simulink model "RobotAndBall"  (R2019b)
settings: Solver=VariableStepAuto  StartTime=0.0  StopTime=30  MaxStep=updateFrequency  RelTol=1e-3
values from neighbouring files (symbols this model uses):
  g = bTraj.GoalOnRight    [Launch_Game_TwoRobots.m]
  pOpponentSidePoint = [2.4;0;0.02]'    [Launch_Game_TwoRobots.m]
  Robot1 = RobotPlayer2(initialQ,TransMat1,DistToTable,'Left')    [Launch_Game_TwoRobots.m]
undefined symbols (not defined in the file or in its folder): Ball, Contact_Forces, currentTime, Environment, Net, Robots, Table, tHit, wayPoints, X, Y, Z
libraries: sm_lib x217, nesl_utility x89, Contact_Forces_Lib x8, robotmaniplib x8, Parts_Lib x6, Multibody_Parts_Lib x2, OpenManipulatorLib x1
(part 7 of 7)

== system RobotAndBall/Subsystem2/Robot 2/Robotic Arm1/iiwa_link_7 ==
  Inertia : sm_lib/Body Elements/Inertia  InertiaType=Custom  Mass=3.129  MassUnits=kg  CenterOfMass=[0, 0, 0]  CenterOfMassUnits=m  MomentsOfInertia=[0.01464, 0.01465, 0.002872]  MomentsOfInertiaUnits=kg*m^2  ProductsOfInertia=[0, 0, 0.0005912]  ProductsOfInertiaUnits=kg*m^2  GraphicType=None  MarkerShape=Inertia  MarkerSize=20  GraphicVisPropType=SimpleVisualProperties  GraphicDiffuseColor=[0.5 0.5 0.5]  GraphicSpecularColor=[0.5 0.5 0.5 1.0]  GraphicAmbientColor=[0.15 0.15 0.15 1.0]  GraphicEmissiveColor=[0.0 0.0 0.0 1.0]  GraphicShininess=75  GraphicOpacity=1.0
  InertiaOriginTransform : sm_lib/Frames and Transforms/Rigid Transform  TranslationMethod=Cartesian  TranslationStandardOffset=0  TranslationLengthUnit=m  TranslationStandardAxis=+Z  TranslationCartesianOffset=[0, 0, 0.02]  TranslationROffset=0  TranslationROffsetUnits=m  TranslationZOffset=0  TranslationZOffsetUnits=m  TranslationThetaOffset=0  TranslationThetaOffsetUnits=deg  RotationMethod=RotationSequence  RotationAngleUnits=deg  RotationStandardAxis=+Z  RotationAngle=0.0  RotationArbitraryAxis=[0 0 1]  FollAlignAxisA=+X  BaseAlignAxisA=+Y  FollAlignAxisB=+Y  BaseAlignAxisB=+Z  RotationSequenceAxes=BaseAxes  RotationSequence=XYZ  RotationSequenceAngles=[0, 0, 0]  RotationSequenceAnglesUnits=rad  RotationMatrix=[1 0 0; 0 1 0; 0 0 1]
  ReferenceFrame : sm_lib/Frames and Transforms/Reference Frame
  Visual : sm_lib/Body Elements/File Solid  ExtGeomFileName=link_7.stl  UnitType=Custom  ExtGeomFileUnits=m  StepReaderType=HEX  ExportEntireGeometry=off  InertiaType=Custom  Mass=0  MassUnits=kg  CenterOfMass=[0, 0, 0]  CenterOfMassUnits=m  MomentsOfInertia=[0, 0, 0]  MomentsOfInertiaUnits=kg*m^2  ProductsOfInertia=[0, 0, 0]  ProductsOfInertiaUnits=kg*m^2  BasedOnType=DensityFromFile  Density=1000  DensityUnits=kg/m^3  DoExposeReferenceFrame=on  SerializedFrames=<Frames/>  GraphicType=FromGeometry  MarkerShape=Sphere  MarkerSize=10  GraphicVisPropType=SimpleVisualProperties  GraphicDiffuseColor=[0.4, 0.4, 0.4]  GraphicSpecularColor=[0.5 0.5 0.5 1.0]  GraphicAmbientColor=[0.15 0.15 0.15 1.0]  GraphicEmissiveColor=[0.0 0.0 0.0 1.0]  GraphicShininess=75  GraphicOpacity=1
  VisualOriginTransform : sm_lib/Frames and Transforms/Rigid Transform  TranslationMethod=Cartesian  TranslationStandardOffset=0  TranslationLengthUnit=m  TranslationStandardAxis=+Z  TranslationCartesianOffset=[0, 0, -0.0005]  TranslationROffset=0  TranslationROffsetUnits=m  TranslationZOffset=0  TranslationZOffsetUnits=m  TranslationThetaOffset=0  TranslationThetaOffsetUnits=deg  RotationMethod=RotationSequence  RotationAngleUnits=deg  RotationStandardAxis=+Z  RotationAngle=0.0  RotationArbitraryAxis=[0 0 1]  FollAlignAxisA=+X  BaseAlignAxisA=+Y  FollAlignAxisB=+Y  BaseAlignAxisB=+Z  RotationSequenceAxes=BaseAxes  RotationSequence=XYZ  RotationSequenceAngles=[0, 0, 0]  RotationSequenceAnglesUnits=rad  RotationMatrix=[1 0 0; 0 1 0; 0 0 1]
  iiwa_joint_7_AxisInvTransform : sm_lib/Frames and Transforms/Rigid Transform  TranslationMethod=Cartesian  TranslationStandardOffset=0  TranslationLengthUnit=m  TranslationStandardAxis=+Z  TranslationCartesianOffset=[0, 0, 0]  TranslationROffset=0  TranslationROffsetUnits=m  TranslationZOffset=0  TranslationZOffsetUnits=m  TranslationThetaOffset=0  TranslationThetaOffsetUnits=deg  RotationMethod=ArbitraryAxis  RotationAngleUnits=rad  RotationStandardAxis=+Z  RotationAngle=0  RotationArbitraryAxis=[1, 0, 0]  FollAlignAxisA=+X  BaseAlignAxisA=+Y  FollAlignAxisB=+Y  BaseAlignAxisB=+Z  RotationSequenceAxes=FollowerAxes  RotationSequence=XYX  RotationSequenceAngles=[0 0 0]  RotationSequenceAnglesUnits=deg  RotationMatrix=[1 0 0; 0 1 0; 0 0 1]
  iiwa_joint_8_AxisInvTransform1 : sm_lib/Frames and Transforms/Rigid Transform  TranslationMethod=Cartesian  TranslationStandardOffset=0  TranslationLengthUnit=m  TranslationStandardAxis=+Z  TranslationCartesianOffset=[0, 0, 0]  TranslationROffset=0  TranslationROffsetUnits=m  TranslationZOffset=0  TranslationZOffsetUnits=m  TranslationThetaOffset=0  TranslationThetaOffsetUnits=deg  RotationMethod=ArbitraryAxis  RotationAngleUnits=rad  RotationStandardAxis=+Z  RotationAngle=0  RotationArbitraryAxis=[0, 0, 1]  FollAlignAxisA=+X  BaseAlignAxisA=+Y  FollAlignAxisB=+Y  BaseAlignAxisB=+Z  RotationSequenceAxes=FollowerAxes  RotationSequence=XYX  RotationSequenceAngles=[0 0 0]  RotationSequenceAnglesUnits=deg  RotationMatrix=[1 0 0; 0 1 0; 0 0 1]
  iiwa_joint_ee_OriginTransform : sm_lib/Frames and Transforms/Rigid Transform  TranslationMethod=Cartesian  TranslationStandardOffset=0  TranslationLengthUnit=m  TranslationStandardAxis=+Z  TranslationCartesianOffset=[0, 0, 0.045]  TranslationROffset=0  TranslationROffsetUnits=m  TranslationZOffset=0  TranslationZOffsetUnits=m  TranslationThetaOffset=0  TranslationThetaOffsetUnits=deg  RotationMethod=RotationSequence  RotationAngleUnits=deg  RotationStandardAxis=+Z  RotationAngle=0.0  RotationArbitraryAxis=[0 0 1]  FollAlignAxisA=+X  BaseAlignAxisA=+Y  FollAlignAxisB=+Y  BaseAlignAxisB=+Z  RotationSequenceAxes=BaseAxes  RotationSequence=XYZ  RotationSequenceAngles=[0, 0, 0]  RotationSequenceAnglesUnits=rad  RotationMatrix=[1 0 0; 0 1 0; 0 0 1]
  F : PMIOPort  Side=Left
  F1 : PMIOPort  Port=2  Side=Right
  connections:
  Inertia/RConn1 -- InertiaOriginTransform/RConn1
  ReferenceFrame/RConn1 -- InertiaOriginTransform/LConn1 -- iiwa_joint_ee_OriginTransform/LConn1 -- iiwa_joint_7_AxisInvTransform/LConn1 -- VisualOriginTransform/LConn1
  Visual/RConn1 -- VisualOriginTransform/RConn1
  iiwa_joint_7_AxisInvTransform/RConn1 -- F/RConn1
  iiwa_joint_8_AxisInvTransform1/RConn1 -- F1/RConn1
  iiwa_joint_ee_OriginTransform/RConn1 -- iiwa_joint_8_AxisInvTransform1/LConn1

== system RobotAndBall/Subsystem2/Robot 2/Robotic Arm1/iiwa_link_8 ==
  Inertia : sm_lib/Body Elements/Inertia  InertiaType=Custom  Mass=0.24*0  MassUnits=kg  CenterOfMass=[0, 0, 0.02]*0  CenterOfMassUnits=m  MomentsOfInertia=[322.661e-6 , 1182.846e-6, 867.899e-6]*0  MomentsOfInertiaUnits=kg*m^2  ProductsOfInertia=[-0.001e-6, 0.002e-6, 0.021e-6]*0  ProductsOfInertiaUnits=kg*m^2  GraphicType=None  MarkerShape=Inertia  MarkerSize=20  GraphicVisPropType=SimpleVisualProperties  GraphicDiffuseColor=[0.5 0.5 0.5]  GraphicSpecularColor=[0.5 0.5 0.5 1.0]  GraphicAmbientColor=[0.15 0.15 0.15 1.0]  GraphicEmissiveColor=[0.0 0.0 0.0 1.0]  GraphicShininess=75  GraphicOpacity=1.0
  Inertia1 : sm_lib/Body Elements/Inertia  Commented=on  InertiaType=Custom  Mass=1000  MassUnits=kg  CenterOfMass=[0, 0, 0.02]  CenterOfMassUnits=m  MomentsOfInertia=1000*[322.661e-6 , 1182.846e-6, 867.899e-6]  MomentsOfInertiaUnits=kg*m^2  ProductsOfInertia=[-0.001e-6, 0.002e-6, 0.021e-6]  ProductsOfInertiaUnits=kg*m^2  GraphicType=None  MarkerShape=Inertia  MarkerSize=20  GraphicVisPropType=SimpleVisualProperties  GraphicDiffuseColor=[0.5 0.5 0.5]  GraphicSpecularColor=[0.5 0.5 0.5 1.0]  GraphicAmbientColor=[0.15 0.15 0.15 1.0]  GraphicEmissiveColor=[0.0 0.0 0.0 1.0]  GraphicShininess=75  GraphicOpacity=1.0
  InertiaOriginTransform : sm_lib/Frames and Transforms/Rigid Transform  TranslationMethod=Cartesian  TranslationStandardOffset=0  TranslationLengthUnit=m  TranslationStandardAxis=+Z  TranslationCartesianOffset=[0, 0,0.05]  TranslationROffset=0  TranslationROffsetUnits=m  TranslationZOffset=0  TranslationZOffsetUnits=m  TranslationThetaOffset=0  TranslationThetaOffsetUnits=deg  RotationMethod=RotationSequence  RotationAngleUnits=deg  RotationStandardAxis=+Z  RotationAngle=0.0  RotationArbitraryAxis=[0 0 1]  FollAlignAxisA=+X  BaseAlignAxisA=+Y  FollAlignAxisB=+Y  BaseAlignAxisB=+Z  RotationSequenceAxes=BaseAxes  RotationSequence=XYZ  RotationSequenceAngles=[0, 0, 0]  RotationSequenceAnglesUnits=rad  RotationMatrix=[1 0 0; 0 1 0; 0 0 1]
  ReferenceFrame : sm_lib/Frames and Transforms/Reference Frame
  Visual : sm_lib/Body Elements/File Solid  ExtGeomFileName=paddle.stl  UnitType=Custom  ExtGeomFileUnits=cm  StepReaderType=HEX  ExportEntireGeometry=off  InertiaType=Custom  Mass=0  MassUnits=kg  CenterOfMass=[0, 0, 0]  CenterOfMassUnits=m  MomentsOfInertia=[0, 0, 0]  MomentsOfInertiaUnits=kg*m^2  ProductsOfInertia=[0, 0, 0]  ProductsOfInertiaUnits=kg*m^2  BasedOnType=DensityFromFile  Density=1000  DensityUnits=kg/m^3  DoExposeReferenceFrame=on  SerializedFrames=<Frames/>  GraphicType=FromGeometry  MarkerShape=Sphere  MarkerSize=10  GraphicVisPropType=SimpleVisualProperties  GraphicDiffuseColor=[1, 0.423529411765, 0.0392156862745]  GraphicSpecularColor=[0.5 0.5 0.5 1.0]  GraphicAmbientColor=[0.15 0.15 0.15 1.0]  GraphicEmissiveColor=[0.0 0.0 0.0 1.0]  GraphicShininess=75  GraphicOpacity=1
  VisualOriginTransform : sm_lib/Frames and Transforms/Rigid Transform  TranslationMethod=Cartesian  TranslationStandardOffset=0  TranslationLengthUnit=m  TranslationStandardAxis=+Z  TranslationCartesianOffset=[0, 0, 0.12]  TranslationROffset=0  TranslationROffsetUnits=m  TranslationZOffset=0  TranslationZOffsetUnits=m  TranslationThetaOffset=0  TranslationThetaOffsetUnits=deg  RotationMethod=RotationSequence  RotationAngleUnits=deg  RotationStandardAxis=+Z  RotationAngle=0.0  RotationArbitraryAxis=[0 0 1]  FollAlignAxisA=+X  BaseAlignAxisA=+Y  FollAlignAxisB=+Y  BaseAlignAxisB=+Z  RotationSequenceAxes=BaseAxes  RotationSequence=XYZ  RotationSequenceAngles=[180, 0, 0]  RotationSequenceAnglesUnits=deg  RotationMatrix=[1 0 0; 0 1 0; 0 0 1]
  iiwa_joint_6_AxisInvTransform : sm_lib/Frames and Transforms/Rigid Transform  TranslationMethod=Cartesian  TranslationStandardOffset=0  TranslationLengthUnit=m  TranslationStandardAxis=+Z  TranslationCartesianOffset=[0, 0, 0]  TranslationROffset=0  TranslationROffsetUnits=m  TranslationZOffset=0  TranslationZOffsetUnits=m  TranslationThetaOffset=0  TranslationThetaOffsetUnits=deg  RotationMethod=ArbitraryAxis  RotationAngleUnits=rad  RotationStandardAxis=+Z  RotationAngle=0  RotationArbitraryAxis=[1, 0, 0]  FollAlignAxisA=+X  BaseAlignAxisA=+Y  FollAlignAxisB=+Y  BaseAlignAxisB=+Z  RotationSequenceAxes=FollowerAxes  RotationSequence=XYX  RotationSequenceAngles=[0 0 0]  RotationSequenceAnglesUnits=deg  RotationMatrix=[1 0 0; 0 1 0; 0 0 1]
  F : PMIOPort  Side=Left
  F1 : PMIOPort  Port=2  Side=Left
  connections:
  iiwa_joint_6_AxisInvTransform/RConn1 -- F/RConn1
  Visual/RConn1 -- F1/RConn1 -- VisualOriginTransform/RConn1
  VisualOriginTransform/LConn1 -- iiwa_joint_6_AxisInvTransform/LConn1 -- InertiaOriginTransform/LConn1 -- ReferenceFrame/RConn1
  Inertia/RConn1 -- InertiaOriginTransform/RConn1

== system RobotAndBall/Subsystem2/Robot 2/Robotic Arm1/world ==
  ReferenceFrame : sm_lib/Frames and Transforms/Reference Frame
  world_iiwa_joint_OriginTransform : sm_lib/Frames and Transforms/Rigid Transform  TranslationMethod=Cartesian  TranslationStandardOffset=0  TranslationLengthUnit=m  TranslationStandardAxis=+Z  TranslationCartesianOffset=[0, 0, 0]  TranslationROffset=0  TranslationROffsetUnits=m  TranslationZOffset=0  TranslationZOffsetUnits=m  TranslationThetaOffset=0  TranslationThetaOffsetUnits=deg  RotationMethod=RotationSequence  RotationAngleUnits=deg  RotationStandardAxis=+Z  RotationAngle=0.0  RotationArbitraryAxis=[0 0 1]  FollAlignAxisA=+X  BaseAlignAxisA=+Y  FollAlignAxisB=+Y  BaseAlignAxisB=+Z  RotationSequenceAxes=BaseAxes  RotationSequence=XYZ  RotationSequenceAngles=[0, 0, 0]  RotationSequenceAnglesUnits=rad  RotationMatrix=[1 0 0; 0 1 0; 0 0 1]
  F : PMIOPort  Side=Left
  F1 : PMIOPort  Port=2  Side=Right
  connections:
  world_iiwa_joint_OriginTransform/LConn1 -- ReferenceFrame/RConn1 -- F/RConn1
  world_iiwa_joint_OriginTransform/RConn1 -- F1/RConn1

== matlab function RobotAndBall/failTryToPredictTraj/MATLAB Function ==
  data: P input; aa output; V input; N input; t input
function aa = fcn(P,V,N,t)
%         if LastV(3)*V(3)<0 & V(3)>0
% %             Ball.N=0;
%                i = i+1
% %             set_param('Table_Ball','SimulationCommand','pause')
%         end
%         Ball.N=Ball.N+1;
%         Ball.Postitions(Ball.N,:)=P;
%         Ball.Velocities(Ball.N,:)=V;
        moments = (0:t/N:t) 
        if(N>5)
            [fitz,Predicted_P] = Traj_Predict(moments,P(1:N,:),N);
        end
        if Ball.N == 150
            figure 
            plot(fitz) ;
            aa = fitz.a
            fitz.b
            fitz.c
        end
%     end


LastP=P;
LastV=V;
y = u;

== matlab function RobotAndBall/Subsystem2/Air_resistance_Force ==
  data: wx input; f output; wy input; wz input; vx input; vy input; vz input; Cd input; Cl input
function f = Air_Resisctance_Force(wx,wy,wz,vx,vy,vz,Cd,Cl)
w = [wx;wy;wz];
v = [vx;vy;vz];
mb = 0.0027; % ball mass = 2.7 gram
% Cd = Environment.AirDrag;%0.141   ; % drag coefficient
% Cl = Environment.Magnus%0.001; % Magnus coefficient
% Cd = 1;
%a = g - Cd*|v|*v + Cl*(w x b)
f = mb*(-Cd*norm(v)*v + Cl*cross(w,v));

== matlab function RobotAndBall/failTryToPredictTraj/Append ==
  data: V input; Vnew input; P input; Pout output; Vout output; Pnew input; N input; Nout output
function [Pout,Vout,Nout]= fcn(V,Vnew,P,Pnew,N)
    Nout=N+1;    
%     Pout = zeros(500,1);
    Vout = V;
    Vout(Nout,:) = Vnew;
    Pout = P;
    Pout(Nout,:) = Pnew;

== matlab function RobotAndBall/Subsystem2/Third_deg_traj/MATLAB Function3 ==
  data: q__ output; q_ output; q output; t input; Ti input; Tf input; qi input; qf input
function [q__,q_,q]= q(t,Ti,Tf,qi,qf)

% if t<1
%     theta(2)=t;
% else
%     theta(2)=1;
% end
% if (t>1)
% theta(1) = t-1;
% end
% if t>2
%     theta(1) = 1;
% end
T = Tf-Ti;
tt = t*ones(7,1);

q = zeros(7,1);
q_ = zeros(7,1);
q__ = zeros(7,1);

q = q + qi + 3*(tt-Ti).^2./T.^2.*(qf -qi) - 2*(tt-Ti).^3./T.^3.*( qf - qi ); 

q_ = q_ + 6*(tt-Ti)./T.^2.*(qf -qi) - 6*(tt-Ti).^2./T.^3.*( qf - qi );

q__ = q__ + 6./T.^2.*(qf -qi) - 12*(tt-Ti)./T.^3.*( qf - qi );

z = zeros(7,1);
q(tt<Ti) = qi(tt<Ti);
q_(tt<Ti) = z(tt<Ti);
q__(tt<Ti) = z(tt<Ti);
q(tt>Tf) = qf(tt>Tf);
q_(tt>Tf) = z(tt>Tf);
q__(tt>Tf) = z(tt>Tf);
%q__=zeros(7,1);
%q_ = zeros(7,1);
end

== matlab function RobotAndBall/Subsystem2/Control_loop1/ M(q)1 ==
  data: q input; M output
function M = calc_M_opt(q)
q1 = q(1);
q2 = q(2);
q3 = q(3);
q4 = q(4);
q5 = q(5);
q6 = q(6);
q7 = q(7);

%CALC_M_OPT
%    M = CALC_M_OPT(Q1,Q2,Q3,Q4,Q5,Q6)

%    This function was generated by the Symbolic Math Toolbox version 8.4.
%    23-Feb-2020 14:32:52
M = calc_M_opt(q1,q2,q3,q4,q5,q6);

% coder.extrinsic('calc_M_opt_mex')
% M = zeros(7);
% M = calc_M_opt_mex(q1,q2,q3,q4,q5,q6);

== matlab function RobotAndBall/Function-Call Subsystem/DesiredHit ==
  data: currentTime input; tHit output; pHit output; paddleOrientHit output; paddleVHit output; predicted_t input; predicted_P input; predicted_V input; N input; idIn input; id output
function [tHit,pHit,paddleOrientHit,paddleVHit,id] = DesiredHit(currentTime,predicted_t,predicted_P,predicted_V,N,idIn)
% the input is vectors of predicted trajectory of the ball, N is the length
%the output are the needed (moments,position, orientation,velocity) of the
%paddle to hit the ball to return it
% first we will try the fixed plane 
BallRadius = 0.02;
znet       = 0.20;
g = -9.81;
cor = 0.72; % racket coefficient of restitution
fixHitplaneX = -0.8;
idx = bSearch(predicted_P(:,1),N,fixHitplaneX);

tHit = predicted_t(idx);
pHit = predicted_P(idx,:)';
Vi = predicted_V(idx,:)';   %the velocity of the ball before the moment of hitting ; if the spinning is taken into account then this vector will be (1x6)

%where to return the ball (a point on the oponent side)
pOponentSide = [0.3 ; -0.6 ; BallRadius] + [ 1 ; 0.6 ; 0 ].*rand(3,1);
zAboveNet = znet + 0.1 + 0.4*rand(1);

% find ball's initial velocity after hit %from primary report 1st year  
zt = [pHit(3); zAboveNet ;pOponentSide(3)];
xt = [pHit(1); 0 ; pOponentSide(1)];
A = [xt.^2 xt [1;1;1]]
Cz = A\zt;

%the ball's initial velocity after hit
vox =  sqrt(g/(2*Cz(1)));
voz = Cz(2)*v0x + g*pHit(1)/v0x;
voy = (pOponentSide(2) - pHit(2)) / (pOponentSide(1) - pHit(1)) * v0x;

%calculating the desired racket velocity
Vo = [vox;voy;voz];
nrd = (Vo-Vi)/norm(Vo-Vi);
vr = (Vo'*nrd + cor*(Vi'*nrd))/(1+cor);
paddleVHit = vr*nrd;

paddleOrientHit=nrd;
id = idIn;

== matlab function RobotAndBall/Subsystem2/Control_loop2/ M(q)1 ==
  data: q input; M output
function M = calc_M_opt(q)
q1 = q(1);
q2 = q(2);
q3 = q(3);
q4 = q(4);
q5 = q(5);
q6 = q(6);
q7 = q(7);

%CALC_M_OPT
%    M = CALC_M_OPT(Q1,Q2,Q3,Q4,Q5,Q6)

%    This function was generated by the Symbolic Math Toolbox version 8.4.
%    23-Feb-2020 14:32:52
M = calc_M_opt(q1,q2,q3,q4,q5,q6);

% coder.extrinsic('calc_M_opt_mex')
% M = zeros(7);
% M = calc_M_opt_mex(q1,q2,q3,q4,q5,q6);

== matlab function RobotAndBall/Subsystem2/Control_loop1/B_C1 ==
  data: q input; BC output; q_ input
function BC = calc_B_C(q,q_)
%CALC_G

% % coder.extrinsic('calc_B_C_codgen_mex')
% % BC = zeros(7,1);
% % BC = calc_B_C_codgen_mex(q,q_)
BC = zeros(7,1);


q_1 = q_(1);
q_2 = q_(2);
q_3 = q_(3);
q_4 = q_(4);
q_5 = q_(5);
q_6 = q_(6);
q_7 = q_(7);
qq_ = [ q_1*q_2;
 q_1*q_3;
 q_1*q_4;
 q_1*q_5;
 q_1*q_6;
 q_1*q_7;
 q_2*q_3;
 q_2*q_4;
 q_2*q_5;
 q_2*q_6;
 q_2*q_7;
 q_3*q_4;
 q_3*q_5;
 q_3*q_6;
 q_3*q_7;
 q_4*q_5;
 q_4*q_6;
 q_4*q_7;
 q_5*q_6;
 q_5*q_7;
 q_6*q_7];
BC = calc_C1_opt(q(1),q(2),q(3),q(4),q(5),q(6))*(q_.*q_);
BC = BC + calc_B_opt(q(1),q(2),q(3),q(4),q(5),q(6))*qq_;

== matlab function RobotAndBall/Subsystem2/Control_loop1/G(q)1 ==
  data: q input; G output
function G = calc_G(q)
%CALC_G
%    G = CALC_G(Q2,Q3,Q4,Q5,Q6,Q7)

%    This function was generated by the Symbolic Math Toolbox version 8.4.
%    22-Feb-2020 01:11:25
%[q1,q2,q3,q4,q5,q6,q7] = q;

% coder.extrinsic('calc_G_opt_mex')

q1 = q(1);
q2 = q(2);
q3 = q(3);
q4 = q(4);
q5 = q(5);
q6 = q(6);
q7 = q(7);
G = calc_G_opt(q2,q3,q4,q5,q6);
% G = zeros(7,1);
% G = calc_G_opt_mex(q2,q3,q4,q5,q6);

== matlab function RobotAndBall/traj_5_order ==
  data: t input; qdd output; traj_Cs input; timeToHit input; qd output; q output
function [qdd,qd,q] = traj_5_order(t,traj_Cs,timeToHit)  
%     persistent i
%     if isempty(i)
%         i=0;
%     end
   
%             if(t>timeToHit && t< timeToHit+0.1)
%                 t=timeToHit;
% %                 tt = [1 t t^2 t^3 t^4 t^5]';
% %                 q = traj_Cs*tt;
% %                 qd = zeros(7,1);
% %                 qdd = zeros(7,1);
% %                 return
%             end
%             if(t<startTime)
%                 t=startTime;
%             end
%             traj_Cs = reshape(Cs,7,6);
            tt = [1 t t^2 t^3 t^4 t^5]';
            q = traj_Cs*tt;
            
            ttd = [0 1 2*t 3*t^2 4*t^3 5*t^4]';
            qd = traj_Cs*ttd;
            
            ttdd = [0 0 2 6*t 12*t^2 20*t^3]';
            qdd = traj_Cs*ttdd;
end

== matlab function RobotAndBall/Subsystem2/Control_loop2/B_C1 ==
  data: q input; BC output; q_ input
function BC = calc_B_C(q,q_)
%CALC_G

% % coder.extrinsic('calc_B_C_codgen_mex')
% % BC = zeros(7,1);
% % BC = calc_B_C_codgen_mex(q,q_)
BC = zeros(7,1);


q_1 = q_(1);
q_2 = q_(2);
q_3 = q_(3);
q_4 = q_(4);
q_5 = q_(5);
q_6 = q_(6);
q_7 = q_(7);
qq_ = [ q_1*q_2;
 q_1*q_3;
 q_1*q_4;
 q_1*q_5;
 q_1*q_6;
 q_1*q_7;
 q_2*q_3;
 q_2*q_4;
 q_2*q_5;
 q_2*q_6;
 q_2*q_7;
 q_3*q_4;
 q_3*q_5;
 q_3*q_6;
 q_3*q_7;
 q_4*q_5;
 q_4*q_6;
 q_4*q_7;
 q_5*q_6;
 q_5*q_7;
 q_6*q_7];
BC = calc_C1_opt(q(1),q(2),q(3),q(4),q(5),q(6))*(q_.*q_);
BC = BC + calc_B_opt(q(1),q(2),q(3),q(4),q(5),q(6))*qq_;

== matlab function RobotAndBall/Subsystem2/Control_loop2/G(q)1 ==
  data: q input; G output
function G = calc_G(q)
%CALC_G
%    G = CALC_G(Q2,Q3,Q4,Q5,Q6,Q7)

%    This function was generated by the Symbolic Math Toolbox version 8.4.
%    22-Feb-2020 01:11:25
%[q1,q2,q3,q4,q5,q6,q7] = q;

% coder.extrinsic('calc_G_opt_mex')

q1 = q(1);
q2 = q(2);
q3 = q(3);
q4 = q(4);
q5 = q(5);
q6 = q(6);
q7 = q(7);
G = calc_G_opt(q2,q3,q4,q5,q6);
% G = zeros(7,1);
% G = calc_G_opt_mex(q2,q3,q4,q5,q6);

== matlab function RobotAndBall/traj_5_order1 ==
  data: t input; qdd output; traj_Cs input; timeToHit input; qd output; q output
function [qdd,qd,q] = traj_5_order(t,traj_Cs,timeToHit)  
%     persistent i
%     if isempty(i)
%         i=0;
%     end
   
%             if(t>timeToHit && t< timeToHit+0.1)
%                 t=timeToHit;
% %                 tt = [1 t t^2 t^3 t^4 t^5]';
% %                 q = traj_Cs*tt;
% %                 qd = zeros(7,1);
% %                 qdd = zeros(7,1);
% %                 return
%             end
%             if(t<startTime)
%                 t=startTime;
%             end
%             traj_Cs = reshape(Cs,7,6);
            tt = [1 t t^2 t^3 t^4 t^5]';
            q = traj_Cs*tt;
            
            ttd = [0 1 2*t 3*t^2 4*t^3 5*t^4]';
            qd = traj_Cs*ttd;
            
            ttdd = [0 0 2 6*t 12*t^2 20*t^3]';
            qdd = traj_Cs*ttdd;
end
